simulink model "points"  (R2016a)
settings: Solver=VariableStepAuto  StartTime=0.0  StopTime=Inf  RelTol=1e-3
libraries: simulink x6
settings Model: Creator=nmd89  LastModifiedBy=nmd89

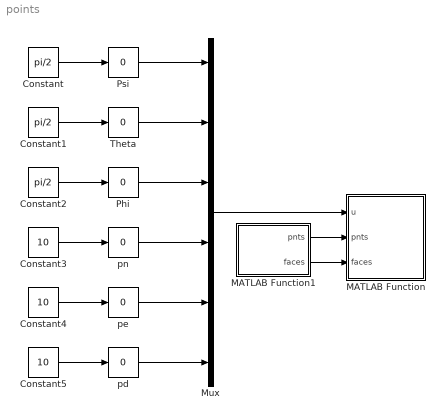
== system points ==
  Constant : Constant  Value=pi/2
  Constant1 : Constant  Value=pi/2
  Constant2 : Constant  Value=pi/2
  Constant3 : Constant  Value=10
  Constant4 : Constant  Value=10
  Constant5 : Constant  Value=10
  MATLAB Function : MATLAB Function  TreatAsAtomicUnit=on
  MATLAB Function1 : MATLAB Function  TreatAsAtomicUnit=on
  Mux : Mux  Inputs=6
  Phi : simulink/Math Operations/Slider Gain  low=-1  gain=0  high=1
  Psi : simulink/Math Operations/Slider Gain  low=-1  gain=0  high=1
  Theta : simulink/Math Operations/Slider Gain  low=-1  gain=0  high=1
  pd : simulink/Math Operations/Slider Gain  low=-1  gain=0  high=1
  pe : simulink/Math Operations/Slider Gain  low=-1  gain=0  high=1
  pn : simulink/Math Operations/Slider Gain  low=-1  gain=0  high=1
  wires:
  Psi/1 -> Mux/1
  Theta/1 -> Mux/2
  Phi/1 -> Mux/3
  Constant/1 -> Psi/1
  Constant1/1 -> Theta/1
  Constant2/1 -> Phi/1
  pn/1 -> Mux/4
  pe/1 -> Mux/5
  pd/1 -> Mux/6
  Constant3/1 -> pn/1
  Constant4/1 -> pe/1
  Constant5/1 -> pd/1
  MATLAB Function1/1(pnts) -> MATLAB Function/2(pnts)
  MATLAB Function1/2(faces) -> MATLAB Function/3(faces)
  Mux/1 -> MATLAB Function/1(u)

== matlab function points/MATLAB Function1 ==
  data: pnts output; faces output
function [pnts, faces] = points()
pnts = [...
    0.25,     0,       0;
    .125,    .1,     -.1;
    .125,   -.1,     -.1;
    .125,   -.1,      .1;
    .125,    .1,      .1;
    -.75,      0,      0;
       0,     .5,      0;
    -.25,     .5,      0;
    -.25,    -.5,      0;
       0,    -.5,      0;
     -.5,    .25,      0;
    -.75,    .25,      0;
    -.75,   -.25,      0;
     -.5,   -.25,      0;
     -.5,      0,      0;
    -.75,      0,    -.25];

faces = [...
    1, 2, 3, NaN;
    1, 3, 4, NaN;
    1, 4, 5, NaN;
    1, 2, 5, NaN;
    3, 4, 6, NaN;
    2, 3, 6, NaN;
    2, 5, 6, NaN;
    4, 5, 6, NaN;
    6, 15, 16, NaN;
    11, 12, 13, 14;
    7, 8, 9, 10];


end

== matlab function points/MATLAB Function ==
  data: u input; pnts input; faces input
function drawAirCraft(u,pnts,faces)
persistent handle 
coder.extrinsic('patch')
psi = u(1);
tht = u(2);
phi = u(3);
pn = u(4);
pe = u(5);
pd = u(6);

% rotate the aircraft
pnts = rotate(pnts',phi,tht,psi);

% translate the aircraft
pnts = translate(pnts',pn,pe,pd);

% transform vertices from NED to XYZ
R = [...
    0,1,0;
    1,0,0;
    0,0,-1];

pnts = pnts*R;

if isempty(handle)
   handle = patch('Vertices',pnts,'Faces',faces,'FaceColor','b');
   axis([-5,5,-5,5,-5,5]);
else
   set(handle,'Vertices',pnts,'Faces',faces);
   axis([pn-1,pn+1,pe-1,pe+1,pd-1,pd+1]);
end
